simulink model "duc"  (R2023b)
settings: Solver=VariableStepAuto  StartTime=0.0  StopTime=0.1  RelTol=1e-3
values from neighbouring files (symbols this model uses):
  bhi = fir2(79,f_l,mhi)    [data_gen.m]
  bhi_h = fir2(79,f_h,mhi)    [data_gen.m]
libraries: dsphdlfiltering2 x3, dspsrcs4 x2, dsphdlsigops2 x1, dspsigops x1
settings Model: Creator=31651  LastModifiedBy=31651

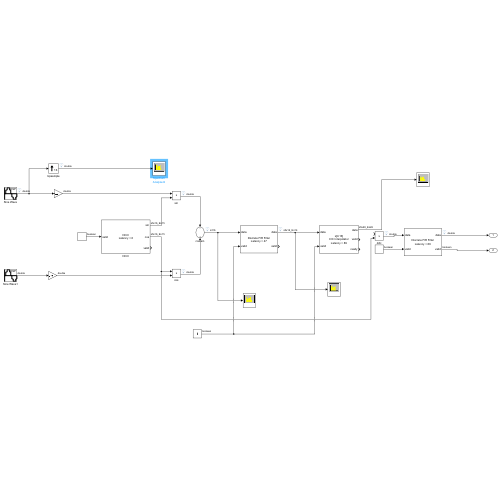
[thumbnail: Simulink's stored preview of the top-level diagram]
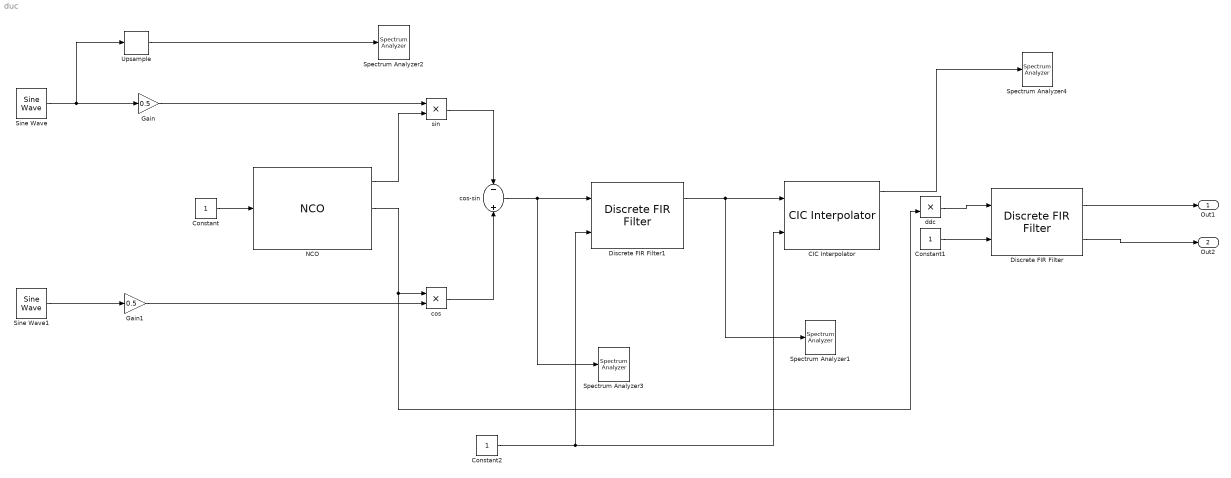
== system duc ==
  CIC Interpolator : dsphdlfiltering2/CIC Interpolator  InterpolationSource=Property  InterpolationFactor=16  MaxInterpolationFactor=2  DifferentialDelay=1  NumSections=4  NumCycles=1  GainCorrection=on  SimulateUsing=Code generation  OutputDataType=Full precision  OutputWordLength=16  ResetInputPort=off  HDLGlobalReset=off
  Constant : Constant  OutDataTypeStr=boolean  SampleTime=1/1000000
  Constant1 : Constant  OutDataTypeStr=boolean  SampleTime=1/1000000
  Constant2 : Constant  OutDataTypeStr=boolean  SampleTime=1/1000000
  Discrete FIR Filter : dsphdlfiltering2/Discrete FIR Filter  NumeratorSource=Property  Numerator=bhi  NumeratorPrototype=[]  FilterStructure=Direct form systolic  SerializationOption=Minimum number of cycles between valid input samples  NumCycles=2  NumberOfMultipliers=2  SimulateUsing=Code generation  roundingMode=Floor  overflowMode=off  CoefficientsDataTypeStr=Inherit: Same word length as input  ResetInputPort=off  HDLGlobalReset=off  CoeffMultiplier=Multiplier  UseMultForPow2Coeff=on
  Discrete FIR Filter1 : dsphdlfiltering2/Discrete FIR Filter  NumeratorSource=Property  Numerator=bhi_h  NumeratorPrototype=[]  FilterStructure=Direct form systolic  SerializationOption=Minimum number of cycles between valid input samples  NumCycles=2  NumberOfMultipliers=2  SimulateUsing=Code generation  roundingMode=Floor  overflowMode=off  CoefficientsDataTypeStr=Inherit: Same word length as input  OutputDataTypeStr=fixdt(1,16,14)  ResetInputPort=off  HDLGlobalReset=off  CoeffMultiplier=Multiplier  UseMultForPow2Coeff=on
  Gain : Gain  Gain=0.5
  Gain1 : Gain  Gain=0.5
  NCO : dsphdlsigops2/NCO  PhaseIncrementSource=Property  PhaseIncrement=6554  PhaseOffsetSource=Property  PhaseOffset=0  DitherSource=Property  NumDitherBits=4  SamplesPerFrame=1  LUTCompress=off  ResetAction=off  Waveform=Sine and cosine  PhasePort=off  SimulateUsing=Code generation  AccumulatorWL=16  PhaseQuantization=on  NumQuantizerAccumulatorBits=12  OutputDataType=Binary point scaling  OutputWL=16  OutputFL=15
      settings: LibrarySourceBlock=dsphdlsrcs2/NCO
  Sine Wave : dspsrcs4/Sine Wave  Amplitude=0.05  Frequency=1000  Phase=0  SampleMode=Discrete  OutComplex=Real  CompMethod=Trigonometric fcn  TableSize=Speed  SampleTime=1/1000000  SamplesPerFrame=1  ResetState=Catch up to simulation time  OutputFrames=off  dataType=double  wordLen=16  udDataType=sfix(16)  fracBitsMode=Best precision  numFracBits=15  OutDataTypeStr=double  LastOutDataTypeStr=double
  Sine Wave1 : dspsrcs4/Sine Wave  Amplitude=0.05  Frequency=1000  Phase=pi/2  SampleMode=Discrete  OutComplex=Real  CompMethod=Trigonometric fcn  TableSize=Speed  SampleTime=1/1000000  SamplesPerFrame=1  ResetState=Catch up to simulation time  OutputFrames=off  dataType=double  wordLen=16  udDataType=sfix(16)  fracBitsMode=Best precision  numFracBits=15  OutDataTypeStr=double  LastOutDataTypeStr=double
  Spectrum Analyzer1 : SpectrumAnalyzer  WindowPosition=[111.000000,166.000000,800.000000,500.000000,]  ScopeFrameLocation=window  Span=99999.99999999999  StartFrequency=-49999.99999999999  StopFrequency=49999.99999999999  YLimits=[-143.3023629,42.5637605]  SelectedToolstripTab=spectrumAnalyzerToolstrip.measurementsTab
  Spectrum Analyzer2 : SpectrumAnalyzer  WindowPosition=[111.000000,166.000000,800.000000,500.000000,]  ScopeFrameLocation=window  Span=99999.99999999999  StartFrequency=-49999.99999999999  StopFrequency=49999.99999999999  YLimits=[-251.48815273,1.78780692]  SelectedToolstripTab=spectrumAnalyzerToolstrip.measurementsTab
  Spectrum Analyzer3 : SpectrumAnalyzer  WindowPosition=[111.000000,166.000000,800.000000,500.000000,]  ScopeFrameLocation=window  Span=99999.99999999999  StartFrequency=-49999.99999999999  StopFrequency=49999.99999999999  YLimits=[-46.05824335,31.7621304]  SelectedToolstripTab=spectrumAnalyzerToolstrip.measurementsTab
  Spectrum Analyzer4 : SpectrumAnalyzer  WindowPosition=[111.000000,166.000000,800.000000,500.000000,]  ScopeFrameLocation=window  Span=99999.99999999999  StartFrequency=-49999.99999999999  StopFrequency=49999.99999999999  YLimits=[-255.1066594,54.91063616]  SelectedToolstripTab=spectrumAnalyzerToolstrip.measurementsTab
  Upsample : dspsigops/Upsample  FactorSource=Dialog parameter  N=16  Nmax=16  phase=0  RateOptions=Allow multirate processing  ic=0  mode=Unused parameter value
      settings: LibrarySourceBlock=dsphdlsupportsigops/Upsample
  cos : Product  OutDataTypeStr=double
  cos-sin : Sum  Inputs=-+  OutDataTypeStr=int16  AccumDataTypeStr=double  LockScale=on
  ddc : Product  OutDataTypeStr=double
  sin : Product  OutDataTypeStr=double
  Out1 : Outport
  Out2 : Outport  Port=2
  wires:
  Constant/1 -> NCO/1
  NCO/1 -> sin/2
  sin/1 -> cos-sin/1
  NCO/2 -> ddc/2, cos/1
  cos/1 -> cos-sin/2
  Sine Wave/1 -> Upsample/1, Gain/1
  Sine Wave1/1 -> Gain1/1
  ddc/1 -> Discrete FIR Filter/1
  Discrete FIR Filter/1 -> Out1/1
  Constant1/1 -> Discrete FIR Filter/2
  Discrete FIR Filter/2 -> Out2/1
  CIC Interpolator/1 -> Spectrum Analyzer4/1
  Constant2/1 -> CIC Interpolator/2, Discrete FIR Filter1/2
  Gain/1 -> sin/1
  Gain1/1 -> cos/2
  cos-sin/1 -> Discrete FIR Filter1/1, Spectrum Analyzer3/1
  Discrete FIR Filter1/1 -> Spectrum Analyzer1/1, CIC Interpolator/1
  Upsample/1 -> Spectrum Analyzer2/1
